simulink model "SkywalkerX8_Observable_Feedback"  (R2018a)
settings: Solver=FixedStepAuto  StartTime=0.0  StopTime=10.0  FixedStep=0.01  RelTol=1e-3
settings Model: Creator=David  LastModifiedBy=David
settings DataIOCC: SaveFormat=StructureWithTime
settings OptimizationCC: BlockReduction=off  BufferReuse=off
settings DebuggingCC: AlgebraicLoopMsg=none  UnconnectedInputMsg=none  UnconnectedOutputMsg=none  UnconnectedLineMsg=none

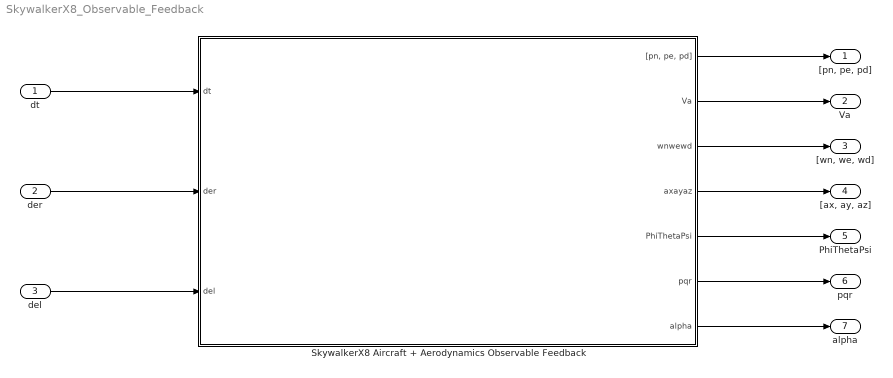
== system SkywalkerX8_Observable_Feedback ==
  dt : Inport
  der : Inport  Port=2
  del : Inport  Port=3
  SkywalkerX8 Aircraft + Aerodynamics Observable Feedback : Subsystem
      mask Display:
      | image('x8SkySunset.png', 'center')
      | 
      | port_label('input', 1, '\delta_t (Unitless)', 'texmode', 'on')
      | port_label('input', 2, '\delta_e_r (rad)', 'texmode', 'on')
      | port_label('input', 3, '\delta_e_l (rad)', 'texmode', 'on')
      | 
      | port_label('output', 1, '[p_N, p_E, p_D] (m)', 'texMode', 'On')
      | port_label('output', 2, 'V_a (m/s)', 'texMode', 'On')
      | port_label('output', 3, '[w_N, w_E, w_D] (m/s)', 'texMode', 'On')
      | port_label('output', 4, '{\bfa_{inertial}} (m/s^2)', 'texMode', 'on')
      | port_label('output', 5, '[\phi, \theta, \psi] (rad)', 'texMode', 'on')
      | port_label('output', 6, '{\bf\omega_b} (rad/s)', 'texMode', 'on')
      | port_label('output', 7, '\alpha (rad)', 'texMode', 'on')
  "[pn, pe, pd]" : Outport
  Va : Outport  Port=2
  "[wn, we, wd]" : Outport  Port=3
  "[ax, ay, az]" : Outport  Port=4
  PhiThetaPsi : Outport  Port=5
  pqr : Outport  Port=6
  alpha : Outport  Port=7
  wires:
  dt/1 -> SkywalkerX8 Aircraft + Aerodynamics Observable Feedback/1(dt)
  der/1 -> SkywalkerX8 Aircraft + Aerodynamics Observable Feedback/2(der)
  del/1 -> SkywalkerX8 Aircraft + Aerodynamics Observable Feedback/3(del)
  SkywalkerX8 Aircraft + Aerodynamics Observable Feedback/1("[pn, pe, pd]") -> "[pn, pe, pd]"/1
  SkywalkerX8 Aircraft + Aerodynamics Observable Feedback/2(Va) -> Va/1
  SkywalkerX8 Aircraft + Aerodynamics Observable Feedback/6(pqr) -> pqr/1
  SkywalkerX8 Aircraft + Aerodynamics Observable Feedback/5(PhiThetaPsi) -> PhiThetaPsi/1
  SkywalkerX8 Aircraft + Aerodynamics Observable Feedback/4(axayaz) -> "[ax, ay, az]"/1
  SkywalkerX8 Aircraft + Aerodynamics Observable Feedback/3(wnwewd) -> "[wn, we, wd]"/1
  SkywalkerX8 Aircraft + Aerodynamics Observable Feedback/7(alpha) -> alpha/1

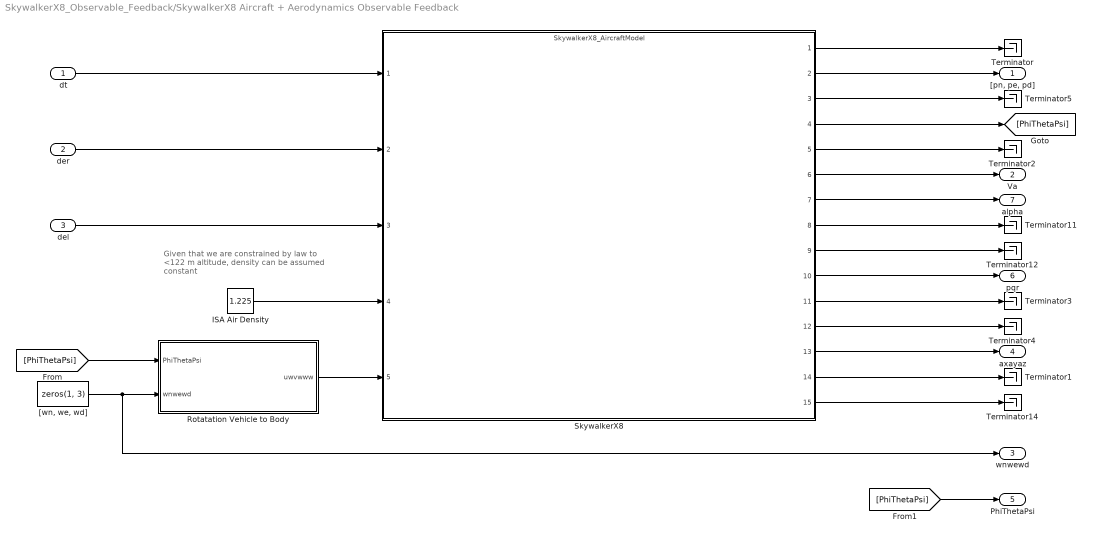
== system SkywalkerX8_Observable_Feedback/SkywalkerX8 Aircraft + Aerodynamics Observable Feedback ==
  note: Given that we are constrained by law to
      | <122 m altitude, density can be assumed
      | constant
  dt : Inport
  der : Inport  Port=2
  del : Inport  Port=3
  ISA Air Density : Constant  Value=1.225
  Rotatation Vehicle to Body : MATLAB Function  TreatAsAtomicUnit=on
  SkywalkerX8 : ModelReference  ModelNameDialog=SkywalkerX8_AircraftModel  ModelReferenceVersion=1.361
      mask Display:
      | image('C:\MATLAB\masters\icons\Skywalker Main Block Icon.png', 'center')
      | 
      | color('cyan')
      | 
      | port_label('input', 1, 'k_{motor} (Unitless)', 'texmode', 'on')
      | port_label('input', 2, '\delta_{er} (rad)', 'texmode', 'on')
      | port_label('input', 3, '\delta_{el} (rad)', 'texmode', 'on')
      | port_label('input', 4, '\rho (kg/m^3)', 'texmode', 'on')
      | port_label('input', 5, '{\bf V_w^b} (m/s)', 'texmode', 'on')
      | 
      | port_label('output', 1, '{\bf V_e} (m/s)', 'texmode', 'on')
      | port_label('output', 2, '{\bf X_e} (m)', 'texmode', 'on')
      | port_label('output', 3, 'Altitude (m)', 'texmode', 'on')
      | port_label('output', 4, '\phi \theta \psi (rad)', 'texmode', 'on')
      | port_label('output', 5, 'R_{inertial}^{body}', 'texmode', 'on')
      | port_label('output', 6, 'V_a (m/s)', 'texmode', 'on')
      | port_label('output', 7, 'alpha (rad)', 'texmode', 'on')
      | port_label('output', 8, 'beta (rad)', 'texmode', 'on')
      | port_label('output', 9, '{\bf V_b} (m/s)', 'texmode', 'on')
      | port_label('output', 10, '{\bf \omega_b} (rad/s)', 'texmode', 'on')
      | port_label('output', 11, '{\bf \delta\omega_b/\deltat} (rad/s^2)', 'texmode', 'on')
      | port_label('output', 12, '{\bf a_{body}} (m/s^2)', 'texmode', 'on')
      | port_label('output', 13, '{\bf a_{inertial}} (m/s^2)', 'texmode', 'on')
      | port_label('output', 14, '\chi (rad)', 'texmode', 'on')
      | port_label('output', 15, '\chi_c (rad)', 'texmode', 'on')
  Terminator{,1..5,11..12,14} (9 alike) : Terminator
  "[wn, we, wd]" : Constant  Value=zeros(1, 3)
  "[pn, pe, pd]" : Outport
  Va : Outport  Port=2
  wnwewd : Outport  Port=3
  axayaz : Outport  Port=4
  PhiThetaPsi : Outport  Port=5
  pqr : Outport  Port=6
  alpha : Outport  Port=7
  wires:
  SkywalkerX8/12 -> Terminator4/1
  SkywalkerX8/13 -> axayaz/1
  Rotatation Vehicle to Body/1(uwvwww) -> SkywalkerX8/5
  SkywalkerX8/11 -> Terminator3/1
  SkywalkerX8/6 -> Va/1
  SkywalkerX8/1 -> Terminator/1
  SkywalkerX8/5 -> Terminator2/1
  SkywalkerX8/7 -> alpha/1
  dt/1 -> SkywalkerX8/1
  SkywalkerX8/8 -> Terminator11/1
  SkywalkerX8/3 -> Terminator5/1
  SkywalkerX8/9 -> Terminator12/1
  SkywalkerX8/2 -> "[pn, pe, pd]"/1
  SkywalkerX8/4 -> [PhiThetaPsi]
  SkywalkerX8/15 -> Terminator14/1
  SkywalkerX8/10 -> pqr/1
  ISA Air Density/1 -> SkywalkerX8/4
  SkywalkerX8/14 -> Terminator1/1
  del/1 -> SkywalkerX8/3
  der/1 -> SkywalkerX8/2
  "[wn, we, wd]"/1 -> wnwewd/1, Rotatation Vehicle to Body/2(wnwewd)
  [PhiThetaPsi] -> Rotatation Vehicle to Body/1(PhiThetaPsi)
  [PhiThetaPsi] -> PhiThetaPsi/1

== matlab function SkywalkerX8_Observable_Feedback/SkywalkerX8 Aircraft + Aerodynamics Observable Feedback/Rotatation Vehicle to Body ==
  data: PhiThetaPsi input; uwvwww output; wnwewd input
function uwvwww = fcn(PhiThetaPsi, wnwewd)

    Phi = PhiThetaPsi(1);
    Theta = PhiThetaPsi(2);
    Psi = PhiThetaPsi(3);

    Rvb = [cos(Theta)*cos(Psi)                             , cos(Theta)*sin(Psi)                             , -sin(Theta)        ;
           sin(Phi)*sin(Theta)*cos(Psi) - cos(Phi)*sin(Psi), sin(Phi)*sin(Theta)*sin(Psi) + cos(Phi)*cos(Psi), sin(Phi)*cos(Theta);
           cos(Phi)*sin(Theta)*cos(Psi) + sin(Phi)*sin(Psi), cos(Phi)*sin(Theta)*sin(Psi) - sin(Phi)*cos(Psi), cos(Phi)*cos(Theta)];

    wnwewed = reshape(wnwewd, 3, 1);

    uwvwww = Rvb*wnwewed;
    
end
